simulink model "Motors_Model_NoPID"  (R2025a)
settings: Solver=VariableStepAuto  StartTime=0.0  StopTime=5  RelTol=1e-3
settings Model: Creator=jjger  LastModifiedBy=jjger

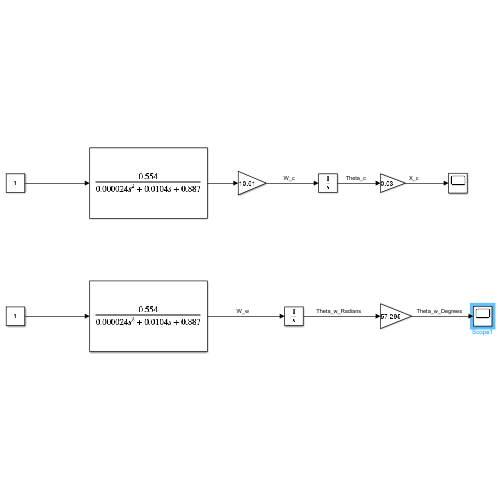
[thumbnail: Simulink's stored preview of the top-level diagram]
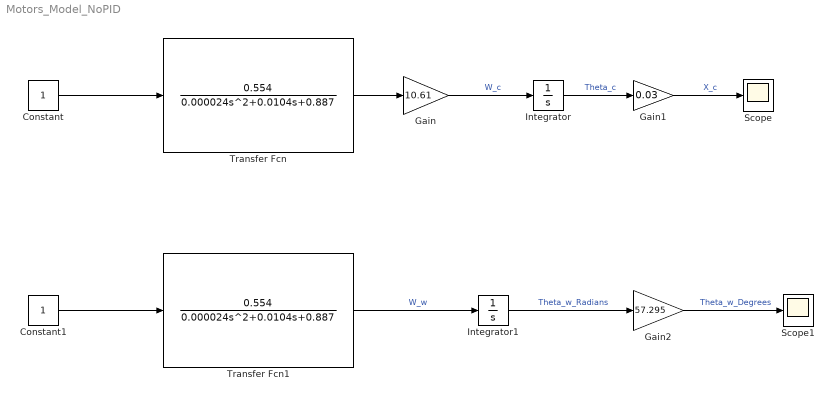
== system Motors_Model_NoPID ==
  Constant : Constant
  Constant1 : Constant
  Gain : Gain  Gain=10.61
  Gain1 : Gain  Gain=0.03
  Gain2 : Gain  Gain=57.295
  Integrator : Integrator
  Integrator1 : Integrator
  Scope : Scope
      settings: ActiveDisplayYMinimum=0.22110873275697129  ActiveDisplayYMaximum=0.71166237622183737
  Scope1 : Scope
      settings: ActiveDisplayYMinimum=-18.815794194996244  ActiveDisplayYMaximum=118.16834420222955
  Transfer Fcn : TransferFcn  Numerator=[0.554]  Denominator=[0.000024 0.0104 0.887]
  Transfer Fcn1 : TransferFcn  Numerator=[0.554]  Denominator=[0.000024 0.0104 0.887]
  wires:
  Constant/1 -> Transfer Fcn/1
  Constant1/1 -> Transfer Fcn1/1
  Transfer Fcn/1 -> Gain/1
  Gain/1 -> Integrator/1  "W_c"
  Integrator/1 -> Gain1/1  "Theta_c"
  Transfer Fcn1/1 -> Integrator1/1  "W_w"
  Gain1/1 -> Scope/1  "X_c"
  Integrator1/1 -> Gain2/1  "Theta_w_Radians"
  Gain2/1 -> Scope1/1  "Theta_w_Degrees"
